simulink model "conversion_type_test"  (R2024b)
settings: Solver=FixedStepDiscrete  StartTime=0.0  StopTime=T  RelTol=1e-12
values from neighbouring files (symbols this model uses):
  Fs = 44100    [Biquad_Test_Filter_v3.m]    (also in Biquad_Test_Filter_v4.m; Biquad_Test_Filter_v4_test.m; Biquad_Test_Filter_v5_test.m = 48000; Biquad_Test_Filter_v6_test.m = 48000)
  x = 2*sin(2*pi*500*t)+1*sin(2*pi*5000*t)    [Biquad_Test_Filter_v3.m]    (also in Biquad_Test_Filter_v4.m = sin(2*pi*1000*t)+sin(2*pi*50*t); Biquad_Test_Filter_v4_test.m = sin(2*pi*1000*t)+sin(2*pi*50*t); Biquad_Test_Filter_v5_test.m = sin(2*pi*1000*t)+sin(2*pi*50*t); Biquad_Test_Filter_v6_test.m = sin(2*pi*1000*t)+sin(2*pi*50*t))
libraries: dspsrcs4 x2
settings Model: DataTypeOverride=Off  Creator=korvo  LastModifiedBy=korvo
settings OptimizationCC: BlockReduction=off  ConditionallyExecuteInputs=off  DefaultParameterBehavior=Inlined  InheritOutputTypeSmallerThanSingle=on
settings DebuggingCC: AlgebraicLoopMsg=error  ArtificialAlgebraicLoopMsg=error  SingleTaskRateTransMsg=error  UnconnectedInputMsg=warning  UnconnectedOutputMsg=warning  UnconnectedLineMsg=warning
settings HardwareCC: ProdBitPerPointer=32  ProdBitPerSizeT=32  ProdBitPerPtrDiffT=32  ProdLargestAtomicFloat=None  ProdIntDivRoundTo=Undefined  ProdEndianess=Unspecified  ProdWordSize=32  ProdHWDeviceType=ASIC/FPGA->ASIC/FPGA  TargetBitPerPointer=64  TargetBitPerSizeT=64  TargetBitPerPtrDiffT=64  TargetLongLongMode=on  TargetIntDivRoundTo=Zero  TargetEndianess=LittleEndian  TargetWordSize=64  TargetHWDeviceType=Custom Processor->MATLAB Host Computer  ProdEqTarget=off

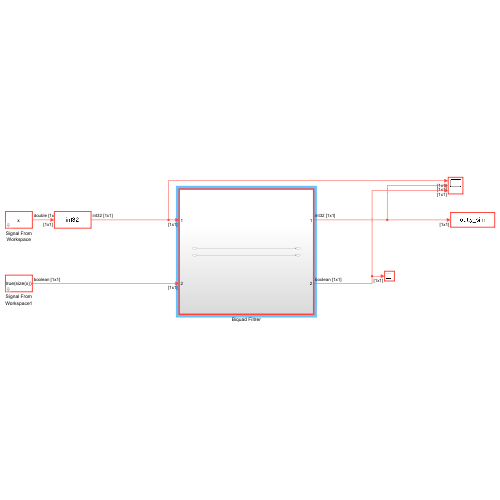
[thumbnail: Simulink's stored preview of the top-level diagram]
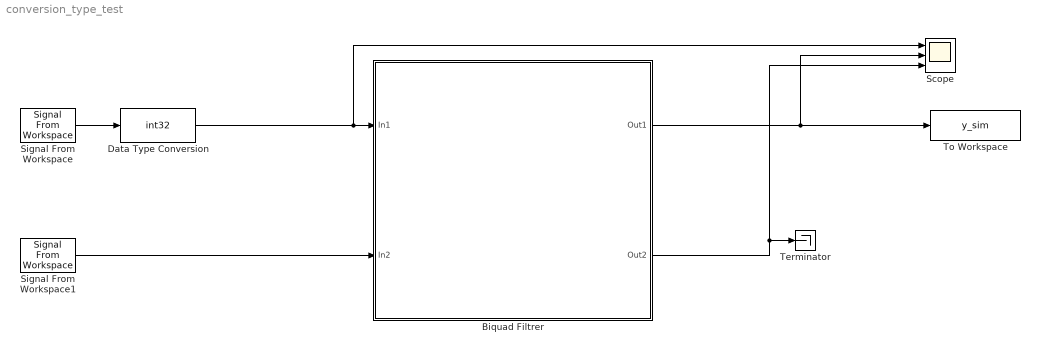
== system conversion_type_test ==
  Biquad Filtrer : Subsystem  TreatAsAtomicUnit=on
  Data Type Conversion : DataTypeConversion  OutDataTypeStr=int32  SaturateOnIntegerOverflow=off  RndMeth=Floor
  Scope : Scope  NumInputPorts=3
  Signal From Workspace : dspsrcs4/Signal From Workspace  X=x  Ts=1/Fs  nsamps=1  OutputAfterFinalValue=Setting to zero  ignoreOrWarnInputAndFrameLengths=off  OutputFrames=off
  Signal From Workspace1 : dspsrcs4/Signal From Workspace  X=true(size(x))  Ts=1/Fs  nsamps=1  OutputAfterFinalValue=Setting to zero  ignoreOrWarnInputAndFrameLengths=off  OutputFrames=off
  Terminator : Terminator
  To Workspace : ToWorkspace  VariableName=y_sim  SampleTime=-1
      settings: Save2DSignal=2-D array (concatenate along first dimension)
  wires:
  Signal From Workspace/1 -> Data Type Conversion/1
  Biquad Filtrer/2(Out2) -> Scope/3, Terminator/1
  Signal From Workspace1/1 -> Biquad Filtrer/2(In2)
  Data Type Conversion/1 -> Scope/1, Biquad Filtrer/1(In1)
  Biquad Filtrer/1(Out1) -> Scope/2, To Workspace/1

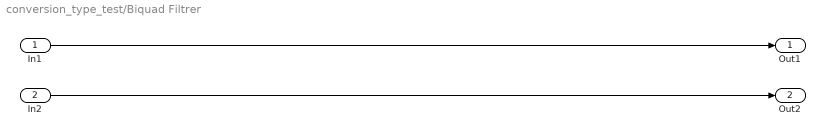
== system conversion_type_test/Biquad Filtrer ==
  In1 : Inport
  In2 : Inport  Port=2
  Out1 : Outport
  Out2 : Outport  Port=2
  wires:
  In2/1 -> Out2/1
  In1/1 -> Out1/1
